simulink model "sdrzWalkieTalkieRx"  (R2016a)
settings: Solver=ode45  StartTime=0.0  StopTime=inf  RelTol=1e-3
PostLoadFcn:
  | sdrzWalkieTalkieRxParams = sdrzWalkieTalkieRxHelper_SimParams();
  | sdrzWalkieTalkieRxHelper_ModelParamsMask('applyParametersToModel');
InitFcn:
  | sdrzWalkieTalkieRxParams = sdrzWalkieTalkieRxHelper_SimParams();
  | sdrzWalkieTalkieRxHelper_ModelParamsMask('applyParametersToModel');
undefined symbols (not defined in the file or in its folder): fdesignblkfcn, gcbh
libraries: dspsnks4 x1, sdrzblksprivate x1, sdrzlib x1, dspmlti4 x1, commrfcorlib x1
CloseFcn:
  | clear sdrzWalkieTalkieRxParams GoertzelCoeffs
Description:
  | This model uses Simulink(R) to receive an FM signal from a suitable commercial walkie-talkie using SDR hardware.
settings Model: SimulationMode=accelerator  Creator=The MathWorks, Inc.  LastModifiedBy=The MathWorks, Inc.
settings DataIOCC: LimitDataPoints=on  SaveFormat=Array
settings DebuggingCC: SolverPrmCheckMsg=warning  ParameterPrecisionLossMsg=none  AllowSymbolicDim=off
settings HardwareCC: ProdBitPerPointer=32  ProdLargestAtomicFloat=None  ProdIntDivRoundTo=Undefined  ProdEndianess=Unspecified  ProdWordSize=32  ProdHWDeviceType=32-bit Generic
settings ModelReferenceCC: PropagateSignalLabelsOutOfModel=off
settings ConfigComp: CovModelRefEnable=Off  CovSFcnEnable=off

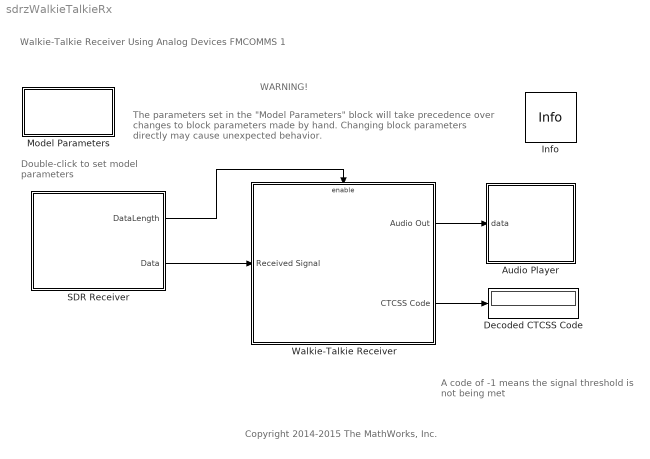
== system sdrzWalkieTalkieRx ==
  note: A code of -1 means the signal threshold
      | is not being met
  note: Walkie-Talkie Receiver Using Analog Devices FMCOMMS 1
  note: Double-click to
      | set model parameters
  note: The parameters set in the "Model Parameters" block will
      | take precedence over changes to block parameters made by hand.
      | Changing block parameters directly may cause unexpected behavior.
  note: WARNING!
  note: Copyright 2014-2015 The MathWorks, Inc.
  Audio Player : Subsystem
  Decoded CTCSS Code : Display
  Info : sdrzblksprivate/Info  SystemSampleTime=-1
  Model Parameters : Subsystem  TreatAsAtomicUnit=on  mask(Model Parameters){walkieTalkieProtocol=FRS, channelFRS=1, channelPMR446=4, CTCSSCode=5, CTCSSDecodeBlockLength=4000, signalPowerThreshold=0.1}
      mask prompts: walkieTalkieProtocol "Walkie-talkie protocol:"; channelFRS "Channel (1 to 14):"; channelPMR446 "Channel (1 to 8):"; CTCSSCode "CTCSS code (0 to 38):"; CTCSSDecodeBlockLength "CTCSS decode block length:"; signalPowerThreshold "Signal threshold for squelch:"
      mask help: Changing these values defines the model parameters needed for reception.
      mask init:
      | sdrzWalkieTalkieRxHelper_ModelParamsMask('applyParametersToModel');
      mask Help: sdrzdemohelp;
      mask TypeOptions walkieTalkieProtocol: FRS | PMR446
      mask Callback walkieTalkieProtocol: sdrzWalkieTalkieRxHelper_ModelParamsMask('maskDisplayUpdate');
      mask Display: disp('Model\nParameters');
  SDR Receiver : Subsystem
  Walkie-Talkie Receiver : Subsystem
  wires:
  Walkie-Talkie Receiver/2(CTCSS Code) -> Decoded CTCSS Code/1
  SDR Receiver/2(Data) -> Walkie-Talkie Receiver/1(Received Signal)
  SDR Receiver/1(DataLength) -> Walkie-Talkie Receiver/Enable
  Walkie-Talkie Receiver/1(Audio Out) -> Audio Player/1(data)

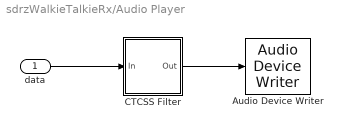
== system sdrzWalkieTalkieRx/Audio Player ==
  data : Inport
  Audio Device Writer : dspsnks4/Audio Device Writer  Driver=DirectSound  Device=Default  InheritSampleRate=on  SampleRate=44100  BitDepth=16-bit integer  BufferSize=4096  NumBuffers=10  DefaultOutputChannelMapping=on  OutputChannelMapping=1:2  OutputNumUnderrunSamples=off  DriverIdx=1  DeviceWarnFlag=''
  CTCSS Filter : Subsystem  DialogController=fdesignblkfcn  InitFcn=fdesignblkfcn(gcbh, {'InitFcn'});  mask(Highpass Filter){}
      mask help: Design a highpass filter
      settings: CopyFcn=fdesignblkfcn(gcbh, {'CopyFcn'});
      mask Help: helpview(mapfilelocation('dsp'), 'dsphighpassfilter');
      mask Display: disp('Highpass')
  wires:
  data/1 -> CTCSS Filter/1(In)
  CTCSS Filter/1(Out) -> Audio Device Writer/1

== system sdrzWalkieTalkieRx/Model Parameters ==
  note: This subsystem is empty.
      | It is used for setting parameter values (in the mask).

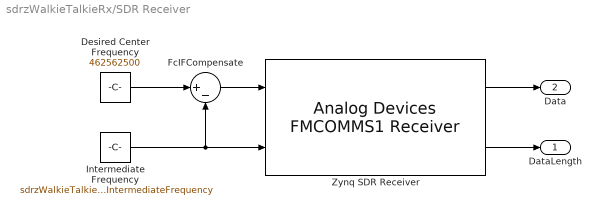
== system sdrzWalkieTalkieRx/SDR Receiver ==
  Desired Center Frequency : Constant  Value=462562500
  FcIFCompensate : Sum  Inputs=|+-
  Intermediate Frequency : Constant  Value=sdrzWalkieTalkieRxParams.radioIntermediateFrequency
  Zynq SDR Receiver : sdrzlib/Analog Devices FMCOMMS1 Receiver  SourceLibraryInfo="This block requires Communications System Toolbox Support Package for Xilinx FPGA-Based Radio. <a href=\"http://www.mathworks.com/hardware-support-packages\">More information</a>"  sobjType=comm.SDRZynqFMCOMMS1Receiver  IPAddress=192.168.3.2  dataUDPPort=-1  ctrlUDPPort=-1  subDeviceList=comm.SDRZynqFMCOMMS1Receiver  sdrBlockType=SDRBlockTypeSLT.SDRRxBlock  requester=UNUSED_BY_SFCN  sdrExecutionMode=HW  LostSamplesOutputPort=off  OutputDataType=single  FrameLength=sdrzWalkieTalkieRxParams.radioFrameSize  EnableBurstMode=off  NumFramesInBurst=20  BypassUserLogic=on  DecimatorSelect=DDC decimator  SourceSelect=RF data  SineAmplitude=16000  SineFrequency=30000  EnableInternalClock=off  BypassIQBalance=on  CenterFrequencySource=Input port  CenterFrequency=2.4e9  IntermediateFrequencySource=Input port  IntermediateFrequency=0  IFBandwidthSource=Dialog  IFBandwidth=40e6  ADCRateSource=Dialog  ADCRate=sdrzWalkieTalkieRxParams.radioADCRate  GainSource=Dialog  Gain=5  DecimationFactorSource=Dialog  DecimationFactor=sdrzWalkieTalkieRxParams.radioDecimationFactor  RFFrequencyIsTunable=logical(1)  SampleTime=sdrzWalkieTalkieRxParams.radioSamplePeriod  BypassDCBlockingFilter=off  IQBalanceCoefficients=64  SkipAllHardwareResetAndInitialization=off  EnableIQCalibrationTable=on  CacheIQCalibrationTable=off
  DataLength : Outport
  Data : Outport  Port=2
  wires:
  FcIFCompensate/1 -> Zynq SDR Receiver/1
  Desired Center Frequency/1 -> FcIFCompensate/1
  Intermediate Frequency/1 -> Zynq SDR Receiver/2, FcIFCompensate/2
  Zynq SDR Receiver/1 -> Data/1
  Zynq SDR Receiver/2 -> DataLength/1

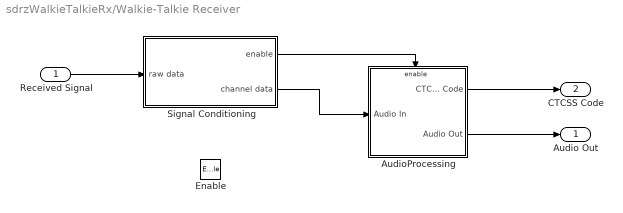
== system sdrzWalkieTalkieRx/Walkie-Talkie Receiver ==
  Received Signal : Inport
  Enable : EnablePort
  AudioProcessing : Subsystem
  Signal Conditioning : Subsystem
  Audio Out : Outport
  CTCSS Code : Outport  Port=2
  wires:
  AudioProcessing/1(CTCSS Code) -> CTCSS Code/1
  Received Signal/1 -> Signal Conditioning/1(raw data)
  Signal Conditioning/1(enable) -> AudioProcessing/Enable
  Signal Conditioning/2(channel data) -> AudioProcessing/1(Audio In)
  AudioProcessing/2(Audio Out) -> Audio Out/1

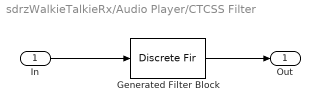
== system sdrzWalkieTalkieRx/Audio Player/CTCSS Filter ==
  In : Inport
  Generated Filter Block : DiscreteFir  Tag=BlockMethodSubSystem  Coefficients=[-0.028925555785371964 -1.1648489870143571e-05 0.00073703943806698632 0.002066323838223116 0.0037924562782123907 0.0058809478036791355 0.0081971633397573667 0.010595694447078679 0.012921336253850104 0.014980443784285901 0.016607828452391647 0.017600625095919989 0.017813808896053544 0.017076060612393459 0.015299380030688972 0.012382878571311963 0.0083283365848107558 0.0031334656085627169 -0.0030917556069984618 -0.010241846567876205 -0.018101550372905492 -0.026471631762265586 -0.035057392286144691 -0.043601476311625496 -0.051774176996057554 -0.059310312221053048 -0.065899215924792212 -0.071322316398364768 -0.075340335280439027 -0.07782838116556251 0.92134179186288967 -0.07782838116556251 -0.075340335280439027 -0.071322316398364768 -0.065899215924792212 -0.059310312221053048 -0.051774176996057554 -0.043601476311625496 -0.035057392286144691 -0.026471631762265586 -0.018101550372905492 -0.010241846567876205 -0.0030917556069984618 0.0031334656085627169 0.0083283365848107558 0.012382878571311963 0.015299380030688972 0.017076060612393459 0.017813808896053544 0.017600625095919989 0.016607828452391647 0.014980443784285901 0.012921336253850104 0.010595694447078679 0.0081971633397573667 0.0058809478036791355 0.0037924562782123907 0.002066323838223116 0.00073703943806698632 -1.1648489870143571e-05 -0.028925555785371964]  InputProcessing=Columns as channels (frame based)
  Out : Outport
  wires:
  In/1 -> Generated Filter Block/1
  Generated Filter Block/1 -> Out/1

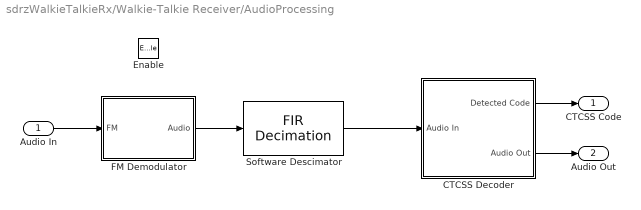
== system sdrzWalkieTalkieRx/Walkie-Talkie Receiver/AudioProcessing ==
  Audio In : Inport
  Enable : EnablePort
  CTCSS Decoder : Subsystem
  FM Demodulator : Subsystem
  Software Descimator : dspmlti4/FIR Decimation  FilterSource=Auto  h=sdrzWalkieTalkieRxParams.decimationCoefficients  D=sdrzWalkieTalkieRxParams.softwareDecimationFactor  filtStruct=Direct form  FilterObject=FDECIM  InputProcessing=Columns as channels (frame based)  framing=Enforce single-rate processing  inputOffset=0  outputBufInitCond=0  roundingMode=Floor  overflowMode=off  firstCoeffDataTypeStr=Inherit: Same word length as input  firstCoeffMin=[]  firstCoeffMax=[]  firstCoeffLastDataTypeStr=Inherit: Same word length as input  outputDataTypeStr=Inherit: Same as accumulator  outputMin=[]  outputMax=[]  outputLastDataTypeStr=Inherit: Same as accumulator
  CTCSS Code : Outport  OutputWhenDisabled=reset  InitialOutput=-1
  Audio Out : Outport  Port=2  OutputWhenDisabled=reset  InitialOutput=0
  wires:
  Software Descimator/1 -> CTCSS Decoder/1(Audio In)
  Audio In/1 -> FM Demodulator/1(FM)
  FM Demodulator/1(Audio) -> Software Descimator/1
  CTCSS Decoder/1(Detected Code) -> CTCSS Code/1
  CTCSS Decoder/2(Audio Out) -> Audio Out/1

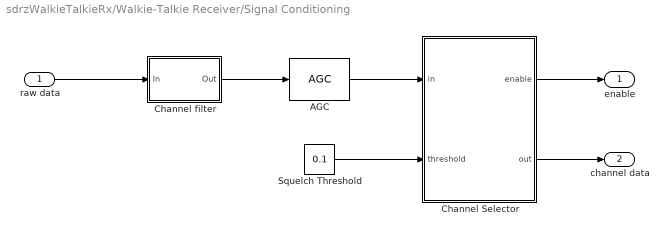
== system sdrzWalkieTalkieRx/Walkie-Talkie Receiver/Signal Conditioning ==
  raw data : Inport
  AGC : commrfcorlib/AGC  LegacyMode=off  DetectorMethod=Rectifier  LoopMethod=Linear  UpdatePeriod=200  StepSize=0.1  AdaptationStepSize=0.01  DesiredOutputPower=1  AveragingLength=100  MaximumGain=1e6  MaxPowerGain=60  GainOutputPort=off  InputPowerOutputPort=off  SimulateUsing=Code generation
  Channel Selector : MATLAB Function  TreatAsAtomicUnit=on
  Channel filter : Subsystem  DialogController=fdesignblkfcn  InitFcn=fdesignblkfcn(gcbh, {'InitFcn'});  mask(Lowpass Filter){}
      mask help: Design a lowpass filter
      settings: CopyFcn=fdesignblkfcn(gcbh, {'CopyFcn'});
      mask Help: helpview(mapfilelocation('dsp'), 'dsplowpassfilter');
      mask Display: disp('Lowpass')
  Squelch Threshold : Constant  Value=0.1  VectorParams1D=off  OutDataTypeStr=single  FramePeriod=-1
  enable : Outport
  channel data : Outport  Port=2
  wires:
  Squelch Threshold/1 -> Channel Selector/2(threshold)
  raw data/1 -> Channel filter/1(In)
  Channel Selector/2(out) -> channel data/1
  Channel Selector/1(enable) -> enable/1
  Channel filter/1(Out) -> AGC/1
  AGC/1 -> Channel Selector/1(in)

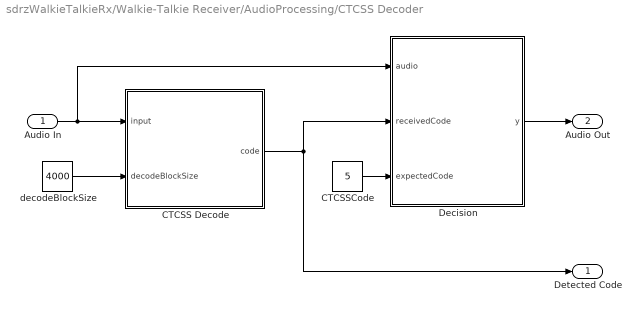
== system sdrzWalkieTalkieRx/Walkie-Talkie Receiver/AudioProcessing/CTCSS Decoder ==
  Audio In : Inport
  CTCSS Decode : MATLAB Function  TreatAsAtomicUnit=on
  CTCSSCode : Constant  Value=5
  Decision : MATLAB Function  TreatAsAtomicUnit=on
  decodeBlockSize : Constant  Value=4000
  Detected Code : Outport
  Audio Out : Outport  Port=2
  wires:
  CTCSSCode/1 -> Decision/3(expectedCode)
  Audio In/1 -> Decision/1(audio), CTCSS Decode/1(input)
  CTCSS Decode/1(code) -> Decision/2(receivedCode), Detected Code/1
  Decision/1(y) -> Audio Out/1
  decodeBlockSize/1 -> CTCSS Decode/2(decodeBlockSize)

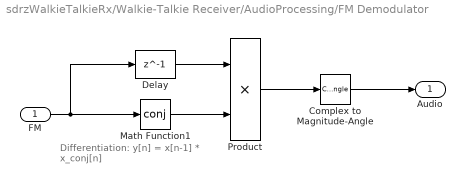
== system sdrzWalkieTalkieRx/Walkie-Talkie Receiver/AudioProcessing/FM Demodulator ==
  note: Differentiation:
      | y[n] = x[n-1] * x_conj[n]
  FM : Inport
  Complex to Magnitude-Angle : ComplexToMagnitudeAngle  Output=Angle
  Delay : Delay  DelayLength=1  InitialCondition=0  InputProcessing=Columns as channels (frame based)
  Math Function1 : Math  Operator=conj  SaturateOnIntegerOverflow=on
  Product : Product  RndMeth=Zero
  Audio : Outport
  wires:
  Complex to Magnitude-Angle/1 -> Audio/1
  Math Function1/1 -> Product/2
  FM/1 -> Math Function1/1, Delay/1
  Delay/1 -> Product/1
  Product/1 -> Complex to Magnitude-Angle/1

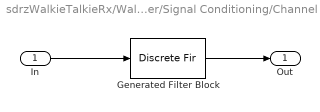
== system sdrzWalkieTalkieRx/Walkie-Talkie Receiver/Signal Conditioning/Channel filter ==
  In : Inport
  Generated Filter Block : DiscreteFir  Tag=BlockMethodSubSystem  FilterStructure=Direct form transposed  Coefficients=[-0.032572119321686695 -0.0075188284161728418 -0.0035638951960136416 0.0031285465646086327 0.010918419520454775 0.017404135429133747 0.020174416990377239 0.0174381774880999 0.0088483279136704149 -0.0042361044317724798 -0.018595166995007035 -0.029997298125918108 -0.033822387278969614 -0.026488112009911607 -0.0064746519625138929 0.025244578821400129 0.06482910993017646 0.10630771786324174 0.14273829721604755 0.16766069504781586 0.17651268744384549 0.16766069504781586 0.14273829721604755 0.10630771786324174 0.06482910993017646 0.025244578821400129 -0.0064746519625138929 -0.026488112009911607 -0.033822387278969614 -0.029997298125918108 -0.018595166995007035 -0.0042361044317724798 0.0088483279136704149 0.0174381774880999 0.020174416990377239 0.017404135429133747 0.010918419520454775 0.0031285465646086327 -0.0035638951960136416 -0.0075188284161728418 -0.032572119321686695]  InputProcessing=Columns as channels (frame based)
  Out : Outport
  wires:
  In/1 -> Generated Filter Block/1
  Generated Filter Block/1 -> Out/1

== matlab function sdrzWalkieTalkieRx/Walkie-Talkie Receiver/Signal Conditioning/Channel Selector ==
  data: in input; enable output; threshold input; out output size=[sdrzWalkieTalkieRxParams.radioFrameSize, 1]
function [enable, out] = squelchFilter(in, threshold)
%#codegen
% Compute the average power of the input signal, if it is greater than a
% threshold, set the enable high, otherwise, low.
out = in;

len = length(in); 
power = sum(abs(in)) / len;

if (power >= threshold)
    enable = true;
else 
    enable = false;
end

== matlab function sdrzWalkieTalkieRx/Walkie-Talkie Receiver/AudioProcessing/CTCSS Decoder/Decision ==
  data: audio input; y output size=[sdrzWalkieTalkieRxParams.radioFrameSize/sdrzWalkieTalkieRxParams.softwareDecimationFactor, 1]; receivedCode input; expectedCode input
function y  = CTCSSCodeCompare(audio, receivedCode, expectedCode)
%#codegen

% If the decoded code equals to pre-specified code, or the pre-specified
% code is 0 (no CTCSS), the audio signal goes through, otherwise, output
% zero.

if ((receivedCode == expectedCode) || (expectedCode == 0))
    y = audio;
else
    y = single(zeros(length(audio),1));
end

== matlab function sdrzWalkieTalkieRx/Walkie-Talkie Receiver/AudioProcessing/CTCSS Decoder/CTCSS Decode ==
  data: input input; code output int8; GoertzelCoeffs parameter; decodeBlockSize input
function code  = CTCSS_Decode(input, GoertzelCoeffs, decodeBlockSize)
%#codegen
% CTCSS decoder for use in a tone squelch system.
%
% Requires identification of one of a set of tones in the audio stream.
% Input is a frame of audio samples at a sample rate of (close to) 8kHz.
%
% Each time the function is called when a frame of samples comes in. It
% changes the state of the function, s(n), s(n-1), s(n-2). When a block of
% samples passes through (block size specified by frs_decodeBlockSize ),
% the power at each frequency is computed by Goertzel algorithm and the
% state is cleared to zero, preparing for the next block. The block size
% could be much larger than the frame size. 
%
% Below is the frequency table for private codes. 
% 
% PL   Hz     PL   Hz      PL   Hz
% --  ----    --  -----    --  -----
%  1  67.0    12  100.0    32  203.5
%  2  71.9    13  103.5    33  210.7
%  3  74.4    14  107.2    34  218.1
%  4  77.0    15  110.9    35  225.7
%  5  79.7    16  114.8    36  233.6
%  6  82.5    17  118.8    37  241.8
%  7  85.4    18  123.0    38  250.3
%  8  88.5    19  127.3
%  9  91.5    20  131.8
% 10  94.8    21  136.5
% 11  97.4    22  141.3
%             23  146.2
%             24  151.4
%             25  156.7
%             26  162.2
%             27  167.9
%             28  173.8
%             29  179.9
%             30  186.2
%             31  192.8
 
nTones = length(GoertzelCoeffs);

persistent  s_d1 s_d2 s maxPowerIdx nProcessed

if isempty(s_d1)
    s_d1 = coder.nullcopy(single(zeros(nTones,1)));% s_d1 = s(n-1)
    s_d2 = coder.nullcopy(single(zeros(nTones,1)));% s_d2 = s(n-2)
    s = coder.nullcopy(single(zeros(nTones,1))); % s = s(n)
    nProcessed = 0;
    maxPowerIdx = 0; 
end

frameSize = length(input);

% The number of sample needs to be processed
nSampleProc = min(frameSize, decodeBlockSize - nProcessed);

for i = 1:nSampleProc
	inputVec = repmat(input(i), nTones,1);
    % s(n) = x(n) + 2cos(2*pi*w)s(n-1) - s(n-2)
	s  = inputVec + GoertzelCoeffs .* s_d1 - s_d2; 
	s_d2 = s_d1;
	s_d1 = s;
end

nProcessed  = nProcessed + nSampleProc;

% if a block is done
if (nProcessed == decodeBlockSize)
	
	power = s_d2.^2 + s_d1.^2 - GoertzelCoeffs .* s_d2 .* s_d1;

    if (any(power ~= 0))
        [~, maxPowerIdx] = max(power);
    end

    % clear the state
	s_d1 = single(zeros(nTones,1));
	s_d2 = single(zeros(nTones,1));
	
    % next block starts, process the remaining samples in the current frame
	for i = nSampleProc + 1 : frameSize
		inputVec = repmat(input(i), nTones,1);
		s  = inputVec + GoertzelCoeffs .* s_d1 - s_d2;
		s_d2 = s_d1;
		s_d1 = s;
	end
	nProcessed = frameSize - nSampleProc;

end

code = int8(maxPowerIdx);
